simulink model "AN_Simulink_Model_v1_fil"  (R2019b)
settings: Solver=VariableStepAuto  StartTime=0.0  StopTime=testtime  RelTol=1e-3
InitFcn:
  | AN_InitFcn_Callback
StopFcn:
  | AN_StopFcn_Callback
values from neighbouring files (symbols this model uses):
  tdres = 1/Fs    (= 2.08333333333e-05)    [AN_Set_Model_Parameters.m]
libraries: hdlmdlgenlib x163, simulink x4, fillib x1, dspsrcs4 x1
(part 5 of 5)

== system AN_Simulink_Model_v1_fil/Auditory Nerve Model/Subsystem/IHC C1 NL Logarithmic Function/Subsystem1/Product3 ==
  In1 : Inport
  In2 : Inport  Port=2
  Product3 : Product  Inputs=**  OutDataTypeStr=single  SampleTime=2.08333333333333e-05
  Out1 : Outport
  wires:
  Product3/1 -> Out1/1
  In2/1 -> Product3/2
  In1/1 -> Product3/1

== system AN_Simulink_Model_v1_fil/Auditory Nerve Model/Subsystem/IHC C1 NL Logarithmic Function/Subsystem1/Product4 ==
  In1 : Inport
  In2 : Inport  Port=2
  Product4 : Product  Inputs=**  OutDataTypeStr=single  SampleTime=2.08333333333333e-05
  Out1 : Outport
  wires:
  Product4/1 -> Out1/1
  In2/1 -> Product4/2
  In1/1 -> Product4/1

== system AN_Simulink_Model_v1_fil/Auditory Nerve Model/Subsystem/IHC C1 NL Logarithmic Function/Subsystem1/Subtract1 ==
  In1 : Inport
  In2 : Inport  Port=2
  Subtract1 : Sum  Inputs=+-  OutDataTypeStr=single  SampleTime=2.08333333333333e-05  SaturateOnIntegerOverflow=on  InputSameDT=on
  Out1 : Outport
  wires:
  Subtract1/1 -> Out1/1
  In2/1 -> Subtract1/2
  In1/1 -> Subtract1/1

== system AN_Simulink_Model_v1_fil/Auditory Nerve Model/Subsystem/IHC C2 NL Logarithmic Function/Subsystem1/Add3 ==
  In1 : Inport
  In2 : Inport  Port=2
  Add3 : Sum  OutDataTypeStr=single  SampleTime=2.08333333333333e-05  SaturateOnIntegerOverflow=on  InputSameDT=on
  Out1 : Outport
  wires:
  Add3/1 -> Out1/1
  In2/1 -> Add3/2
  In1/1 -> Add3/1

== system AN_Simulink_Model_v1_fil/Auditory Nerve Model/Subsystem/IHC C2 NL Logarithmic Function/Subsystem1/Divide1 ==
  In1 : Inport
  In2 : Inport  Port=2
  Divide1 : Product  Inputs=*/  OutDataTypeStr=single  SampleTime=2.08333333333333e-05  SaturateOnIntegerOverflow=on  RndMeth=Zero
  Out1 : Outport
  wires:
  Divide1/1 -> Out1/1
  In2/1 -> Divide1/2
  In1/1 -> Divide1/1

== system AN_Simulink_Model_v1_fil/Auditory Nerve Model/Subsystem/IHC C2 NL Logarithmic Function/Subsystem1/Divide2 ==
  In1 : Inport
  In2 : Inport  Port=2
  Divide2 : Product  Inputs=*/  OutDataTypeStr=single  SampleTime=2.08333333333333e-05  SaturateOnIntegerOverflow=on  RndMeth=Zero
  Out1 : Outport
  wires:
  Divide2/1 -> Out1/1
  In2/1 -> Divide2/2
  In1/1 -> Divide2/1

== system AN_Simulink_Model_v1_fil/Auditory Nerve Model/Subsystem/IHC C2 NL Logarithmic Function/Subsystem1/Divide4 ==
  In1 : Inport
  In2 : Inport  Port=2
  Divide4 : Product  Inputs=*/  OutDataTypeStr=single  SampleTime=2.08333333333333e-05  SaturateOnIntegerOverflow=on  RndMeth=Zero
  Out1 : Outport
  wires:
  Divide4/1 -> Out1/1
  In2/1 -> Divide4/2
  In1/1 -> Divide4/1

== system AN_Simulink_Model_v1_fil/Auditory Nerve Model/Subsystem/IHC C2 NL Logarithmic Function/Subsystem1/Divide5 ==
  In1 : Inport
  In2 : Inport  Port=2
  Divide5 : Product  Inputs=*/  OutDataTypeStr=single  SampleTime=2.08333333333333e-05  SaturateOnIntegerOverflow=on  RndMeth=Zero
  Out1 : Outport
  wires:
  Divide5/1 -> Out1/1
  In2/1 -> Divide5/2
  In1/1 -> Divide5/1

== system AN_Simulink_Model_v1_fil/Auditory Nerve Model/Subsystem/IHC C2 NL Logarithmic Function/Subsystem1/Gain2_unaryminus ==
  In1 : Inport
  Gain2_unaryminus : UnaryMinus  SampleTime=2.08333333333333e-05
  Out1 : Outport
  wires:
  Gain2_unaryminus/1 -> Out1/1
  In1/1 -> Gain2_unaryminus/1

== system AN_Simulink_Model_v1_fil/Auditory Nerve Model/Subsystem/IHC C2 NL Logarithmic Function/Subsystem1/Log10 ==
  In1 : Inport
  Log10 : Math  Operator=log10  SampleTime=2.08333333333333e-05  SaturateOnIntegerOverflow=on
  Out1 : Outport
  wires:
  Log10/1 -> Out1/1
  In1/1 -> Log10/1

== system AN_Simulink_Model_v1_fil/Auditory Nerve Model/Subsystem/IHC C2 NL Logarithmic Function/Subsystem1/Math Function1 ==
  In1 : Inport
  Math Function1 : Math  SampleTime=2.08333333333333e-05  SaturateOnIntegerOverflow=on
  Out1 : Outport
  wires:
  Math Function1/1 -> Out1/1
  In1/1 -> Math Function1/1

== system AN_Simulink_Model_v1_fil/Auditory Nerve Model/Subsystem/IHC C2 NL Logarithmic Function/Subsystem1/Product3 ==
  In1 : Inport
  In2 : Inport  Port=2
  Product3 : Product  Inputs=**  OutDataTypeStr=single  SampleTime=2.08333333333333e-05
  Out1 : Outport
  wires:
  Product3/1 -> Out1/1
  In2/1 -> Product3/2
  In1/1 -> Product3/1

== system AN_Simulink_Model_v1_fil/Auditory Nerve Model/Subsystem/IHC C2 NL Logarithmic Function/Subsystem1/Product4 ==
  In1 : Inport
  In2 : Inport  Port=2
  Product4 : Product  Inputs=**  OutDataTypeStr=single  SampleTime=2.08333333333333e-05
  Out1 : Outport
  wires:
  Product4/1 -> Out1/1
  In2/1 -> Product4/2
  In1/1 -> Product4/1

== system AN_Simulink_Model_v1_fil/Auditory Nerve Model/Subsystem/IHC C2 NL Logarithmic Function/Subsystem1/Subtract1 ==
  In1 : Inport
  In2 : Inport  Port=2
  Subtract1 : Sum  Inputs=+-  OutDataTypeStr=single  SampleTime=2.08333333333333e-05  SaturateOnIntegerOverflow=on  InputSameDT=on
  Out1 : Outport
  wires:
  Subtract1/1 -> Out1/1
  In2/1 -> Subtract1/2
  In1/1 -> Subtract1/1

== matlab function AN_Simulink_Model_v1_fil/Compare/Assert_ihcout/RelErrCheck/RelativeErrorCheck  ==
  data: P input; y output; R input; ToleranceValue parameter double
% Check if the relative error of R with respect to P is below
% ToleranceValue
% P, R are floating-point
function y = relErrCheck(P,R, ToleranceValue)
    tol = ToleranceValue;
    sz = numel(P);
    assert(sz == numel(R), 'Inputs P and R have different sizes.');
    y = false(1, sz);

    for ii=1:sz
        if (isnan(P(ii)) || isnan(R(ii)))
            if (isnan(P(ii)) && isnan(R(ii)))
                y(ii) = true;
            end
        elseif (isinf(P(ii)) || isinf(R(ii)))
            y(ii) = (P(ii) == R(ii));
        elseif (P(ii) == 0)
            y(ii) = (R(ii) == 0);
        else
            absdiff = abs(P(ii) - R(ii));
            relerr = absdiff/abs(P(ii));
            y(ii) = (relerr <= tol);
        end
    end
end
